simulink model "PWMlength"  (Simulink 8.8)
settings: Solver=FixedStepDiscrete  StartTime=0.0  StopTime=0.3  RelTol=1e-3
libraries: simulink x2, slrtlib x1
settings Model: Creator=jays  LastModifiedBy=jays  ExtModeTrigDuration=5
settings DataIOCC: LimitDataPoints=off  SaveFormat=Dataset  SignalLoggingSaveFormat=Dataset
settings OptimizationCC: LifeSpan=auto  MaxStackSize=64
settings DebuggingCC: UnderspecifiedInitializationDetection=Simplified  MergeDetectMultiDrivingBlocksExec=error  ParameterTunabilityLossMsg=error  FcnCallInpInsideContextMsg=error  StateNameClashWarn=none  SFUnexpectedBacktrackingDiag=error  SFNoUnconditionalDefaultTransitionDiag=error  SFExecutionAtInitializationDiag=warning
settings HardwareCC: ProdLargestAtomicInteger=Long  ProdLargestAtomicFloat=Double  ProdIntDivRoundTo=Zero  ProdEndianess=LittleEndian  ProdHWDeviceType=ARM Compatible->ARM Cortex
settings ModelReferenceCC: PropagateSignalLabelsOutOfModel=on
settings RTWCC: SystemTargetFile=ert.tlc  HardwareBoard=NXP FRDM-KL25Z  TLCOptions=-aInlineSetEventsForThisBaseRateFcn=TLC_FALSE -aSuppressMultiTaskScheduler=TLC_FALSE -aRateBasedStepFcn=1  TemplateMakefile=ert_default_tmf  Description=Embedded Coder  GenerateReport=on  Toolchain=GNU Tools for ARM Embedded Processors  IncludeHyperlinkInReport=on  LaunchReport=on  GenerateTraceInfo=on  GenerateTraceReport=on  GenerateTraceReportSl=on  GenerateTraceReportSf=on  GenerateTraceReportEml=on
settings MATStruct: className=codertarget.tools.BuildHook  argsTopModelOnly=[]  excludedModels=[]  includeReferencedModels=on  includeTopModel=on  enabled=on  UseCoderTarget=[1]  TargetHardware=Freescale FRDM-KL25Z  RTOS=Baremetal  Scheduler_interrupt_source=[0.0]  DataVersion=2016.02  Baudrate=codertarget.freedomboard.internal.uartActionCallback  COMPort=codertarget.freedomboard.internal.getExternalSerialPortName  Verbose=[1]  Configuration=Serial  Select_UART=[0.0]  BuildAction=Build, load and run  cpuClockRateMHz=48  SCL_Pin=PTB0  SDA_Pin=PTB1  Frequency=4166  BaudRate=115200  Tx_PinSelection=PTA2 (USBTX)  Rx_PinSelection=PTA1 (USBRX)
settings CodeAppCC: ForceParamTrailComments=on  IgnoreCustomStorageClasses=off  OperatorAnnotations=on  SimulinkDataObjDesc=on  SFDataObjDesc=on  MATLABFcnDesc=on  InsertBlockDesc=on  MATLABSourceComments=on
settings ERTTargetCC: MultiwordLength=2048
settings ConfigComp: CovMetricSettings=dwe  CovHtmlReporting=off  CovSaveCumulativeToWorkspaceVar=off  CovSaveSingleToWorkspaceVar=off  CovExternalEMLEnable=on

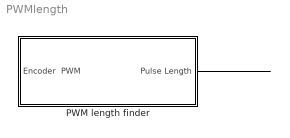
== system PWMlength ==
  PWM length finder : Subsystem
  wires:
  PWM length finder/1(Pulse Length) -> ?
  ? -> PWM length finder/1(Encoder  PWM)

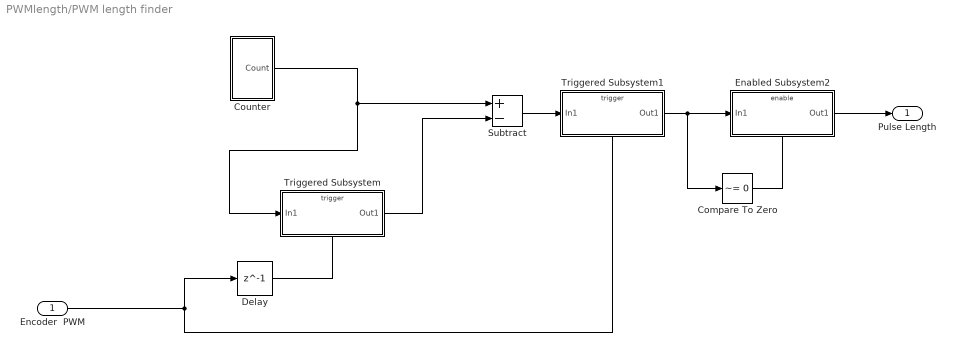
== system PWMlength/PWM length finder ==
  Encoder  PWM : Inport
  Compare To Zero : simulink/Logic and Bit Operations/Compare To Zero  relop=~=  OutDataTypeStr=boolean
  "Counter " : Subsystem
  Delay : Delay  DelayLength=1  InitialCondition=0  SampleTime=0.00001
  Enabled Subsystem2 : Subsystem  TreatAsAtomicUnit=on
  Subtract : Sum  Inputs=+-
  Triggered Subsystem : Subsystem  TreatAsAtomicUnit=on
  Triggered Subsystem1 : Subsystem  TreatAsAtomicUnit=on
  Pulse Length : Outport
  wires:
  Subtract/1 -> Triggered Subsystem1/1(In1)
  "Counter "/1(Count) -> Triggered Subsystem/1(In1), Subtract/1
  Triggered Subsystem/1(Out1) -> Subtract/2
  Triggered Subsystem1/1(Out1) -> Enabled Subsystem2/1(In1), Compare To Zero/1
  Enabled Subsystem2/1(Out1) -> Pulse Length/1
  Compare To Zero/1 -> Enabled Subsystem2/Enable
  Encoder  PWM/1 -> Triggered Subsystem1/Trigger, Delay/1
  Delay/1 -> Triggered Subsystem/Trigger

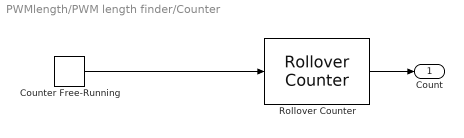
== system PWMlength/PWM length finder/Counter  ==
  Counter Free-Running : simulink/Sources/Counter Free-Running  NumBits=16  tsamp=0.001
  "Rollover Counter " : slrtlib/Incremental Encoder/Utilities/Rollover/Rollover Counter   InitialValue=0  RolloverThreshold=2^15
  Count : Outport
  wires:
  "Rollover Counter "/1 -> Count/1
  Counter Free-Running/1 -> "Rollover Counter "/1

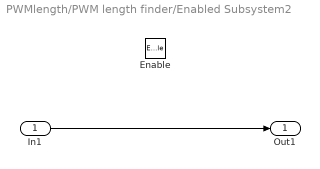
== system PWMlength/PWM length finder/Enabled Subsystem2 ==
  In1 : Inport
  Enable : EnablePort
  Out1 : Outport
  wires:
  In1/1 -> Out1/1

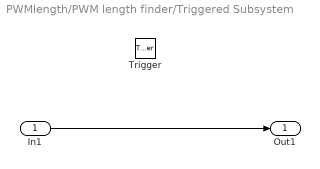
== system PWMlength/PWM length finder/Triggered Subsystem ==
  In1 : Inport
  Trigger : TriggerPort  VariantControl=Variant
  Out1 : Outport
  wires:
  In1/1 -> Out1/1

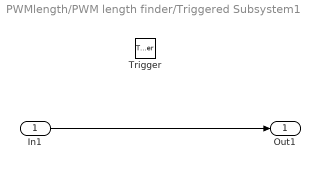
== system PWMlength/PWM length finder/Triggered Subsystem1 ==
  In1 : Inport
  Trigger : TriggerPort  VariantControl=Variant
  Out1 : Outport
  wires:
  In1/1 -> Out1/1
